simulink model "EasyGlider_ManualMode_with_waypoints_and_sysID"  (R2018b)
settings: Solver=FixedStepDiscrete  StartTime=0.0  StopTime=1000  FixedStep=cntrl.sample_time  RelTol=1e-4
values from neighbouring files (symbols this model uses):
  K_pitch = ndiFeedbackGainPlace(-0.5*ones(2,1), 0)    [init_EasyGlider_MM_waypoint_and_sysID.m]
  K_roll = ndiFeedbackGainPlace(-0.5*ones(2,1), 0)    [init_EasyGlider_MM_waypoint_and_sysID.m]
  K_thurst = ndiFeedbackGainPlace(-0.5*ones(2,1), 0)    [init_EasyGlider_MM_waypoint_and_sysID.m]
  K_yaw = ndiFeedbackGainPlace(-0.5*ones(2,1), 0)    [init_EasyGlider_MM_waypoint_and_sysID.m]
  signals_size = length(signals)    [init_EasyGlider_MM_waypoint_and_sysID.m]
  trim_speed = 14    [init_EasyGlider_MM_waypoint_and_sysID.m]
undefined symbols (not defined in the file or in its folder): DiscIntNeverNeededParam, signals
libraries: unit_conversions_lib x3, ardupilot_custom_controller_lib x2, traj_lib x2, rangefinders_lib x1, simulink x1, filters_lib x1
settings Model: DataTypeOverride=Single  DataTypeOverrideAppliesTo=Floating-point  Creator=Yannic  LastModifiedBy=eike
settings SolverCC: ZeroCrossControl=DisableAll
settings DataIOCC: LimitDataPoints=on  SaveOutput=off  SaveTime=off  ReturnWorkspaceOutputs=on
settings OptimizationCC: DefaultParameterBehavior=Inlined  UseDivisionForNetSlopeComputation=on  UseFloatMulNetSlope=on  DefaultUnderspecifiedDataType=single  InlineInvariantSignals=on  PassReuseOutputArgsAs=Individual arguments  ZeroExternalMemoryAtStartup=off  ZeroInternalMemoryAtStartup=off  NoFixptDivByZeroProtection=on  EfficientFloat2IntCast=on  LifeSpan=1  OptimizeBlockOrder=speed  DifferentSizesBufferReuse=on
settings DebuggingCC: ReadBeforeWriteMsg=DisableAll  WriteAfterWriteMsg=DisableAll  WriteAfterReadMsg=DisableAll  MultiTaskDSMMsg=none  ParameterPrecisionLossMsg=none  ParameterTunabilityLossMsg=error  AllowSymbolicDim=off  LibraryContextMissingDiagnostic=none  SFUnexpectedBacktrackingDiag=warning  SFNoUnconditionalDefaultTransitionDiag=warning  SFExecutionAtInitializationDiag=none
settings HardwareCC: ProdBitPerLong=64  ProdLongLongMode=on  ProdHWDeviceType=Intel->x86-64 (Linux 64)
settings ModelReferenceCC: UpdateModelReferenceTargets=IfOutOfDate  PropagateSignalLabelsOutOfModel=off
settings SFSimCC: SFSimEcho=off  SimUseLocalCustomCode=off  MATLABDynamicMemAlloc=off
settings RTWCC: SystemTargetFile=ert.tlc  GenCodeOnly=on  TemplateMakefile=ert_default_tmf  GenerateReport=on  RTWUseLocalCustomCode=off  IncludeHyperlinkInReport=on  LaunchReport=on  TargetLang=C++  GenerateTraceInfo=on  GenerateTraceReport=on  GenerateTraceReportSl=on  GenerateTraceReportSf=on  GenerateTraceReportEml=on
settings CodeAppCC: ForceParamTrailComments=on  IgnoreCustomStorageClasses=off  OperatorAnnotations=on  SimulinkDataObjDesc=on  SFDataObjDesc=on  CustomSymbolStrGlobalVar=rt$N$M  CustomSymbolStrType=$N$M  CustomSymbolStrFcn=$N$M$F  CustomSymbolStrMacro=$N$M  InsertBlockDesc=on
settings ERTTargetCC: TargetLangStandard=C++03 (ISO)  IncludeMdlTerminateFcn=off  CombineSignalStateStructs=on  SuppressErrorStatus=on  SupportAbsoluteTime=off  MultiInstanceERTCode=on  CodeInterfacePackaging=C++ class  SupportNonFinite=off  SupportVariableSizeSignals=on  ERTHeaderFileRootName=MatlabController$E  ERTSourceFileRootName=MatlabController$E  ERTDataFileRootName=MatlabController_data  InlinedParameterPlacement=NonHierarchical  RootIOFormat=Structure reference  ERTCustomFileTemplate=example_file_process.tlc  ERTFilePackagingFormat=CompactWithDataFile
settings ConfigComp: CovMetricSettings=dw  CovHtmlReporting=on  CovSaveCumulativeToWorkspaceVar=on  CovSaveSingleToWorkspaceVar=on  CovExternalEMLEnable=off

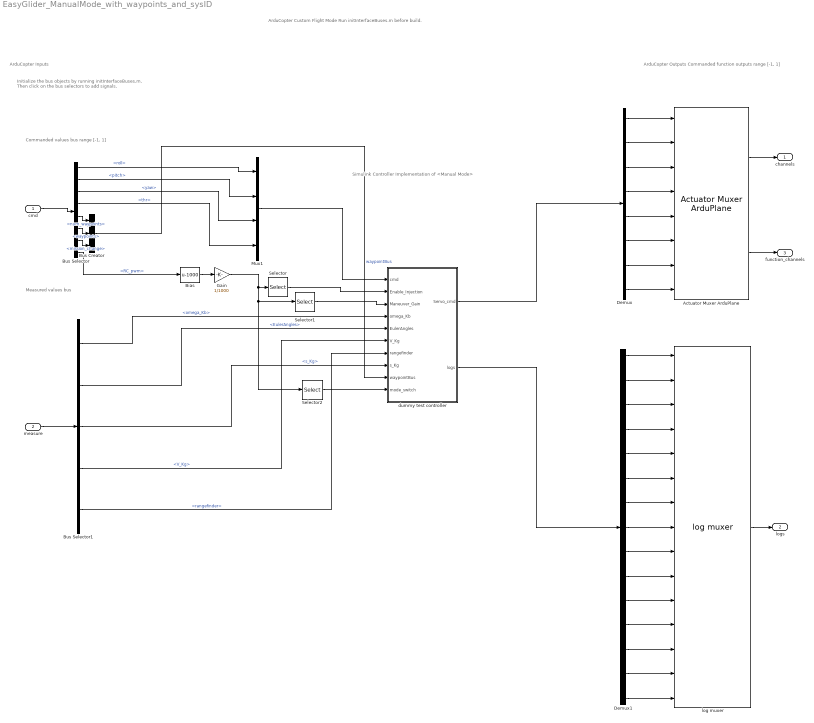
== system EasyGlider_ManualMode_with_waypoints_and_sysID ==
  note: Measured values bus
  note: Initialize the bus objects by running initInterfaceBuses.m.
      | Then click on the bus selectors to add signals.
  note: Commanded values bus
      | range [-1, 1]
  note: ArduCopter Inputs
  note: ArduCopter Outputs
      | Commanded function outputs
      | range [-1, 1]
  note: Simulink Controller
      | Implementation of
      | <Manual Mode>
  note: ArduCopter Custom Flight Mode
      | Run initInterfaceBuses.m before build.
  cmd : Inport  OutDataTypeStr=Bus: cmdBus
  measure : Inport  Port=2  OutDataTypeStr=Bus: measureBus
  Actuator Muxer ArduPlane : ardupilot_custom_controller_lib/Actuator Muxer ArduPlane  CHFCN1=k_aileron  CHFCN2=k_elevator  CHFCN3=k_throttle  CHFCN4=k_rudder  CHFCN5=k_none  CHFCN6=k_none  CHFCN7=k_none  CHFCN8=k_none
      settings: SourceProductName=LADAC
  Bias : Bias  Bias=-1000
  Bus Creator : BusCreator  Inputs=3
  Bus Selector : BusSelector  OutputSignals=roll,pitch,yaw,thr,num_waypoints,waypoints,mission_change,RC_pwm
  Bus Selector1 : BusSelector  OutputSignals=omega_Kb,EulerAngles,s_Kg,V_Kg,rangefinder
  Demux : Demux  Outputs=8
  Demux1 : Demux  Outputs=15
  Gain : Gain  Gain=1/1000
  Mux1 : Mux
  Selector : Selector  InputPortWidth=16  IndexOptions=Index vector (dialog)  Indices=6  OutputSizes=1
  Selector1 : Selector  InputPortWidth=16  IndexOptions=Index vector (dialog)  Indices=7  OutputSizes=1
  Selector2 : Selector  InputPortWidth=16  IndexOptions=Index vector (dialog)  Indices=8  OutputSizes=1
  dummy test controller : Subsystem  DataTypeOverride=Single  DataTypeOverrideAppliesTo=Floating-point
  log muxer : ardupilot_custom_controller_lib/log muxer
      settings: SourceProductName=LADAC
  channels : Outport  OutDataTypeStr=single  PortDimensions=[8]
  logs : Outport  Port=2  OutDataTypeStr=single
  function_channels : Outport  Port=3  OutDataTypeStr=uint16  PortDimensions=[8]
  wires:
  cmd/1 -> Bus Selector/1
  measure/1 -> Bus Selector1/1
  Bus Selector1/2 -> dummy test controller/5(EulerAngles)  "<EulerAngles>"
  Bus Selector1/1 -> dummy test controller/4(omega_Kb)  "<omega_Kb>"
  Bus Selector/1 -> Mux1/1  "<roll>"
  Bus Selector/2 -> Mux1/2  "<pitch>"
  Bus Selector/3 -> Mux1/3  "<yaw>"
  Bus Selector/4 -> Mux1/4  "<thr>"
  Mux1/1 -> dummy test controller/1(cmd)
  Actuator Muxer ArduPlane/1 -> channels/1
  Bus Selector1/4 -> dummy test controller/6(V_Kg)  "<V_Kg>"
  log muxer/1 -> logs/1
  Demux/8 -> Actuator Muxer ArduPlane/8
  Demux/7 -> Actuator Muxer ArduPlane/7
  Demux/6 -> Actuator Muxer ArduPlane/6
  Demux/5 -> Actuator Muxer ArduPlane/5
  Demux/4 -> Actuator Muxer ArduPlane/4
  Demux/3 -> Actuator Muxer ArduPlane/3
  Demux/2 -> Actuator Muxer ArduPlane/2
  Demux/1 -> Actuator Muxer ArduPlane/1
  Demux1/1 -> log muxer/1
  Demux1/2 -> log muxer/2
  Demux1/3 -> log muxer/3
  Demux1/4 -> log muxer/4
  Demux1/5 -> log muxer/5
  Demux1/6 -> log muxer/6
  Demux1/7 -> log muxer/7
  Demux1/8 -> log muxer/8
  Demux1/9 -> log muxer/9
  Demux1/10 -> log muxer/10
  Demux1/11 -> log muxer/11
  Demux1/12 -> log muxer/12
  Demux1/13 -> log muxer/13
  dummy test controller/2(logs) -> Demux1/1
  Bus Selector1/5 -> dummy test controller/7(rangefinder)  "<rangefinder>"
  Actuator Muxer ArduPlane/2 -> function_channels/1
  dummy test controller/1(Servo_cmd) -> Demux/1
  Demux1/14 -> log muxer/14
  Demux1/15 -> log muxer/15
  Bus Selector/6 -> Bus Creator/2  "<waypoints>"
  Bus Selector/5 -> Bus Creator/1  "<num_waypoints>"
  Bus Selector/7 -> Bus Creator/3  "<mission_change>"
  Bus Creator/1 -> dummy test controller/9(waypointBus)  "waypointBus"
  Bus Selector1/3 -> dummy test controller/8(s_Kg)  "<s_Kg>"
  Bus Selector/8 -> Bias/1  "<RC_pwm>"
  Selector/1 -> dummy test controller/2(Enable_Injection)
  Selector1/1 -> dummy test controller/3(Maneuver_Gain)
  Bias/1 -> Gain/1
  Gain/1 -> Selector2/1, Selector1/1, Selector/1
  Selector2/1 -> dummy test controller/10(mode_switch)

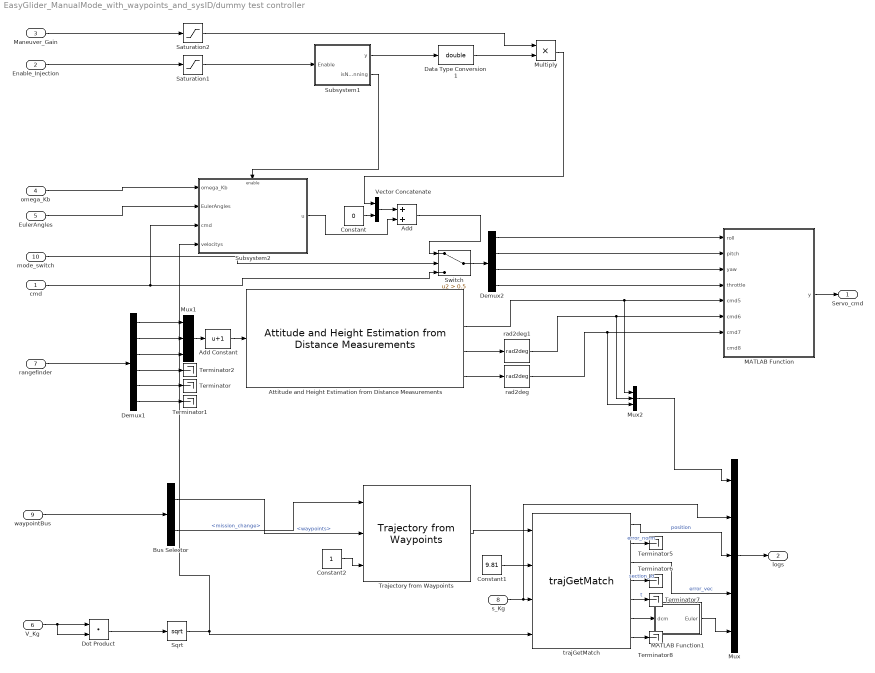
== system EasyGlider_ManualMode_with_waypoints_and_sysID/dummy test controller ==
  cmd : Inport
  Enable_Injection : Inport  Port=2
  Maneuver_Gain : Inport  Port=3
  omega_Kb : Inport  Port=4
  EulerAngles : Inport  Port=5
  V_Kg : Inport  Port=6
  rangefinder : Inport  Port=7
  s_Kg : Inport  Port=8
  waypointBus : Inport  Port=9
  mode_switch : Inport  Port=10
  Add : Sum
  Add Constant : Bias  Bias=1
  Attitude and Height Estimation from Distance Measurements : rangefinders_lib/Attitude and Height Estimation from Distance Measurements  theta=[-75 -75 -75]  psi=[0 90 -90]
  Bus Selector : BusSelector  OutputSignals=waypoints,mission_change
  Constant : Constant  Value=0
  Constant1 : Constant  Value=9.81
  Constant2 : Constant
  Data Type Conversion1 : DataTypeConversion  OutDataTypeStr=double
  Demux1 : Demux  Outputs=6
  Demux2 : Demux
  Dot Product : DotProduct  InputSameDT=on  OutDataTypeStr=Inherit: Inherit via internal rule
  MATLAB Function : MATLAB Function  TreatAsAtomicUnit=on
  MATLAB Function1 : MATLAB Function  TreatAsAtomicUnit=on
  Multiply : Product
  Mux : Mux  Inputs=5
  Mux1 : Mux  Inputs=3
  Mux2 : Mux  Inputs=3
  Saturation1 : Saturate  UpperLimit=1  LowerLimit=0
  Saturation2 : Saturate  UpperLimit=1  LowerLimit=0
  Sqrt : Sqrt  SaturateOnIntegerOverflow=on
  Subsystem1 : Subsystem
  Subsystem2 : Subsystem
  Switch : Switch  Criteria=u2 > Threshold  Threshold=0.5
  Terminator{,1..2,5..8} (7 alike) : Terminator
  Trajectory from Waypoints : traj_lib/Trajectory from Waypoints  traj_params=traj_parms
      settings: SourceProductName=LADAC
  Vector Concatenate : Concatenate
  rad2deg : unit_conversions_lib/rad2deg
      settings: SourceProductName=LADAC
  rad2deg1 : unit_conversions_lib/rad2deg
      settings: SourceProductName=LADAC
  trajGetMatch : traj_lib/trajGetMatch  SystemSampleTime=-1
      settings: SourceProductName=LADAC
  Servo_cmd : Outport
  logs : Outport  Port=2
  wires:
  Mux/1 -> logs/1
  Demux2/1 -> MATLAB Function/1(roll)
  Demux2/2 -> MATLAB Function/2(pitch)
  Demux2/3 -> MATLAB Function/3(yaw)
  cmd/1 -> Subsystem2/3(cmd), Switch/3
  MATLAB Function/1(y) -> Servo_cmd/1
  rangefinder/1 -> Demux1/1
  Demux1/5 -> Terminator/1
  Demux1/6 -> Terminator1/1
  Demux1/1 -> Mux1/1
  Demux1/2 -> Mux1/2
  Demux1/3 -> Mux1/3
  Demux1/4 -> Terminator2/1
  Mux1/1 -> Add Constant/1
  Attitude and Height Estimation from Distance Measurements/3 -> rad2deg1/1
  Attitude and Height Estimation from Distance Measurements/4 -> rad2deg/1
  rad2deg1/1 -> Mux2/2, MATLAB Function/6(cmd6)
  rad2deg/1 -> Mux2/3, MATLAB Function/7(cmd7)
  Attitude and Height Estimation from Distance Measurements/2 -> Mux2/1, MATLAB Function/5(cmd5)
  Bus Selector/2 -> Trajectory from Waypoints/1  "<mission_change>"
  Bus Selector/1 -> Trajectory from Waypoints/2  "<waypoints>"
  Constant1/1 -> trajGetMatch/2
  EulerAngles/1 -> Subsystem2/2(EulerAngles)
  omega_Kb/1 -> Subsystem2/1(omega_Kb)
  waypointBus/1 -> Bus Selector/1
  Add Constant/1 -> Attitude and Height Estimation from Distance Measurements/1
  Trajectory from Waypoints/1 -> trajGetMatch/1
  s_Kg/1 -> Mux/2, trajGetMatch/3
  Sqrt/1 -> Subsystem2/4("velocitys "), trajGetMatch/4
  trajGetMatch/1 -> Mux/3  "position"
  trajGetMatch/2 -> Terminator5/1  "error_norm"
  trajGetMatch/4 -> Terminator6/1  "section_id"
  trajGetMatch/5 -> Terminator7/1  "t"
  trajGetMatch/7 -> Terminator8/1
  trajGetMatch/3 -> Mux/4  "error_vec"
  Subsystem1/1(y) -> Data Type Conversion1/1
  Saturation1/1 -> Subsystem1/1(Enable)
  Maneuver_Gain/1 -> Saturation2/1
  Multiply/1 -> Vector Concatenate/1
  Saturation2/1 -> Multiply/1
  Enable_Injection/1 -> Saturation1/1
  Data Type Conversion1/1 -> Multiply/2
  Subsystem1/2(isNotRunning) -> Subsystem2/Enable
  Add/1 -> Switch/1
  Subsystem2/1(u) -> Add/2
  Dot Product/1 -> Sqrt/1
  V_Kg/1 -> Dot Product/2, Dot Product/1
  Constant2/1 -> Trajectory from Waypoints/3
  trajGetMatch/6 -> MATLAB Function1/1(dcm)
  MATLAB Function1/1(Euler) -> Mux/5
  Mux2/1 -> Mux/1
  Demux2/4 -> MATLAB Function/4(throttle)
  Switch/1 -> Demux2/1
  Vector Concatenate/1 -> Add/1
  Constant/1 -> Vector Concatenate/2
  mode_switch/1 -> Switch/2

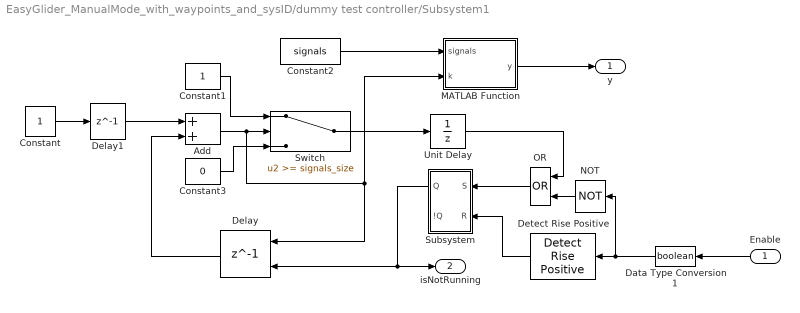
== system EasyGlider_ManualMode_with_waypoints_and_sysID/dummy test controller/Subsystem1 ==
  Enable : Inport
  Add : Sum
  Constant : Constant
  Constant1 : Constant  OutDataTypeStr=boolean
  Constant2 : Constant  Value=signals  VectorParams1D=off
  Constant3 : Constant  Value=0  OutDataTypeStr=boolean
  Data Type Conversion1 : DataTypeConversion  OutDataTypeStr=boolean
  Delay : Delay  DelayLength=1  InitialCondition=1  ExternalReset=Level hold
      settings: InputPortMap=u0,r5
  Delay1 : Delay  DelayLength=1
  Detect Rise Positive : simulink/Logic and Bit Operations/Detect Rise Positive  vinit=0  OutDataTypeStr=boolean
  MATLAB Function : MATLAB Function  TreatAsAtomicUnit=on
  NOT : Logic  Operator=NOT  IconShape=distinctive  AllPortsSameDT=off  OutDataTypeStr=boolean
  OR : Logic  Operator=OR  IconShape=distinctive  AllPortsSameDT=off  OutDataTypeStr=boolean
  Subsystem : Subsystem
  Switch : Switch  Threshold=signals_size
  Unit Delay : UnitDelay  SampleTime=-1
  y : Outport
  isNotRunning : Outport  Port=2
  wires:
  Constant/1 -> Delay1/1
  Delay1/1 -> Add/1
  Delay/1 -> Add/2
  Constant1/1 -> Switch/1
  MATLAB Function/1(y) -> y/1
  Constant2/1 -> MATLAB Function/1(signals)
  Add/1 -> Switch/2, MATLAB Function/2(k), Delay/1
  Subsystem/1(Q) -> isNotRunning/1, Delay/2
  Switch/1 -> Unit Delay/1
  Enable/1 -> Data Type Conversion1/1
  Constant3/1 -> Switch/3
  Data Type Conversion1/1 -> NOT/1, Detect Rise Positive/1
  Unit Delay/1 -> OR/1
  NOT/1 -> OR/2
  OR/1 -> Subsystem/1(S)
  Detect Rise Positive/1 -> Subsystem/2(R)

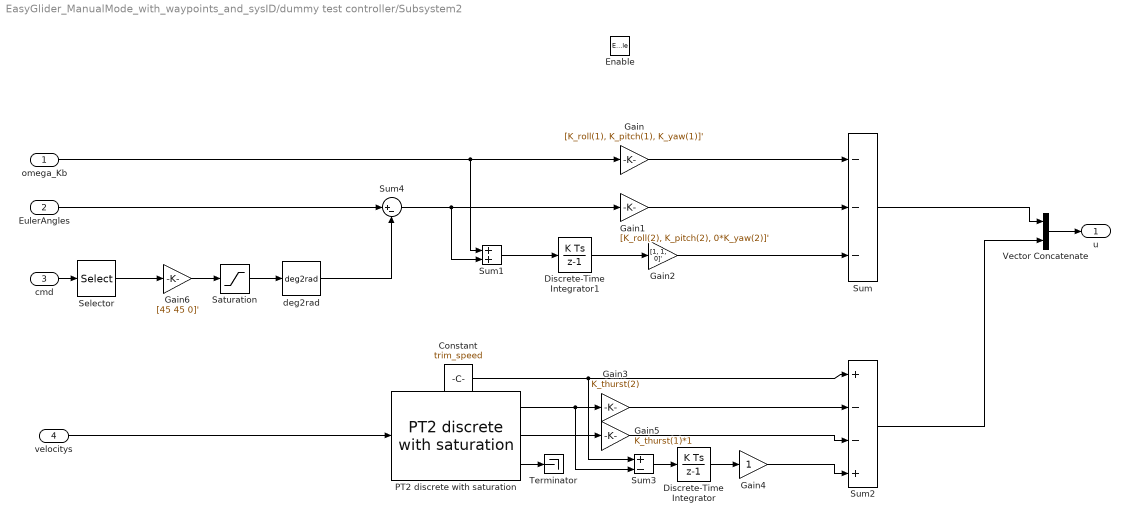
== system EasyGlider_ManualMode_with_waypoints_and_sysID/dummy test controller/Subsystem2 ==
  omega_Kb : Inport
  EulerAngles : Inport  Port=2
  cmd : Inport  Port=3
  "velocitys " : Inport  Port=4
  Enable : EnablePort
  Constant : Constant  Value=trim_speed
  Discrete-Time Integrator : DiscreteIntegrator  SampleTime=-1  LimitOutput=on  UpperSaturationLimit=0.8  LowerSaturationLimit=0  ICPrevOutput=DiscIntNeverNeededParam  ICPrevScaledInput=DiscIntNeverNeededParam
  Discrete-Time Integrator1 : DiscreteIntegrator  SampleTime=-1  ICPrevOutput=DiscIntNeverNeededParam  ICPrevScaledInput=DiscIntNeverNeededParam
  Gain : Gain  Gain=[K_roll(1), K_pitch(1), K_yaw(1)]'
  Gain1 : Gain  Gain=[K_roll(2), K_pitch(2), 0*K_yaw(2)]'
  Gain2 : Gain  Gain=[1, 1, 0]'
  Gain3 : Gain  Gain=K_thurst(2)
  Gain4 : Gain
  Gain5 : Gain  Gain=K_thurst(1)*1
  Gain6 : Gain  Gain=[45 45 0]'
  PT2 discrete with saturation : filters_lib/PT2 discrete with saturation  omega=10  d=1  x_dt2_max=inf  x_dt2_min=-inf  x_dt_max=inf  x_dt_min=-inf  x_max=inf  x_min=-inf  x_init=trim_speed  x_dt_init=0
      settings: SourceProductName=LADAC
  Saturation : Saturate  UpperLimit=45  LowerLimit=-45
  Selector : Selector  InputPortWidth=4  IndexOptions=Index vector (dialog)  Indices=[1 2 3]  OutputSizes=1
  Sum : Sum  Inputs=---
  Sum1 : Sum
  Sum2 : Sum  Inputs=+--+
  Sum3 : Sum  Inputs=+-
  Sum4 : Sum  Inputs=|+-
  Terminator : Terminator
  Vector Concatenate : Concatenate
  deg2rad : unit_conversions_lib/deg2rad
      settings: SourceProductName=LADAC
  u : Outport
  wires:
  Sum/1 -> Vector Concatenate/1
  Sum1/1 -> Discrete-Time Integrator1/1
  omega_Kb/1 -> Sum1/1, Gain/1
  Gain/1 -> Sum/1
  Gain1/1 -> Sum/2
  Discrete-Time Integrator1/1 -> Gain2/1
  Gain2/1 -> Sum/3
  Sum4/1 -> Sum1/2, Gain1/1
  Sum2/1 -> Vector Concatenate/2
  Vector Concatenate/1 -> u/1
  Gain4/1 -> Sum2/4
  Constant/1 -> Sum3/1, Sum2/1
  "velocitys "/1 -> PT2 discrete with saturation/1
  PT2 discrete with saturation/1 -> Sum3/2, Gain3/1
  Gain3/1 -> Sum2/2
  PT2 discrete with saturation/2 -> Gain5/1
  Gain5/1 -> Sum2/3
  Sum3/1 -> Discrete-Time Integrator/1
  Discrete-Time Integrator/1 -> Gain4/1
  PT2 discrete with saturation/3 -> Terminator/1
  cmd/1 -> Selector/1
  Selector/1 -> Gain6/1
  Gain6/1 -> Saturation/1
  Saturation/1 -> deg2rad/1
  EulerAngles/1 -> Sum4/1
  deg2rad/1 -> Sum4/2

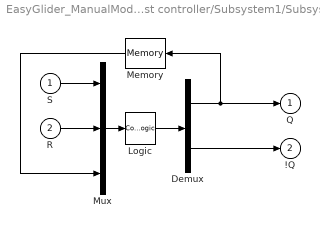
== system EasyGlider_ManualMode_with_waypoints_and_sysID/dummy test controller/Subsystem1/Subsystem ==
  S : Inport
  R : Inport  Port=2
  Demux : Demux  Outputs=2
  Logic : CombinatorialLogic  TruthTable=[0 1;1 0;0 1;0 1;1 0;1 0;1 0;1 0]
  Memory : Memory  InitialCondition=1
  Mux : Mux  Inputs=3
  Q : Outport  InitialOutput=0
  !Q : Outport  Port=2  InitialOutput=1
  wires:
  R/1 -> Mux/2
  S/1 -> Mux/1
  Demux/2 -> !Q/1
  Logic/1 -> Demux/1
  Memory/1 -> Mux/3
  Demux/1 -> Q/1, Memory/1
  Mux/1 -> Logic/1

== matlab function EasyGlider_ManualMode_with_waypoints_and_sysID/dummy test controller/Subsystem1/MATLAB Function ==
  data: signals input; y output; k input
function y = fcn(signals, k)

y = signals(k,1:3)';

end

== matlab function EasyGlider_ManualMode_with_waypoints_and_sysID/dummy test controller/MATLAB Function ==
  data: roll input; y output; pitch input; yaw input; throttle input; cmd5 input; cmd6 input; cmd7 input; cmd8 input
function y = fcn(roll,pitch,yaw,throttle,cmd5,cmd6,cmd7,cmd8)

y = single(zeros(8,1));

y(1) = roll;
y(2) = pitch;
y(3) = throttle;
y(4) = yaw;
y(5) = cmd5 ;
y(6) = cmd6 ;
y(7) = cmd7 ;
y(8) = cmd8 ;

end

== matlab function EasyGlider_ManualMode_with_waypoints_and_sysID/dummy test controller/MATLAB Function1 ==
  data: dcm input; Euler output
function Euler = dcm3Euler(dcm)

Euler = dcm2Euler(dcm);
